simulink model "ImageBasedMdlv2"  (Simulink 9.1)
settings: Solver=VariableStepAuto  StartTime=0.0  StopTime=10.0  RelTol=1e-3
settings Model: Creator=admin  LastModifiedBy=admin
settings DataIOCC: SaveFormat=Dataset
settings OptimizationCC: LifeSpan=auto
settings DebuggingCC: UnderspecifiedInitializationDetection=Simplified  MergeDetectMultiDrivingBlocksExec=error  SFUnexpectedBacktrackingDiag=error  SFNoUnconditionalDefaultTransitionDiag=error  SFExecutionAtInitializationDiag=warning
settings HardwareCC: ProdBitPerPointer=64  ProdBitPerSizeT=64  ProdBitPerPtrDiffT=64  ProdLargestAtomicFloat=Float  ProdIntDivRoundTo=Zero  ProdEndianess=LittleEndian  ProdWordSize=64  ProdHWDeviceType=Intel->x86-64 (Windows64)
settings ModelReferenceCC: PropagateSignalLabelsOutOfModel=on
settings CodeAppCC: StateflowObjectComments=off
settings GRTTargetCC: TargetLangStandard=C99 (ISO)  CombineOutputUpdateFcns=on  GRTInterface=off
settings ConfigComp: CovMetricSettings=dwe  CovHtmlReporting=off  CovSaveCumulativeToWorkspaceVar=off  CovSaveSingleToWorkspaceVar=off  CovExternalEMLEnable=on

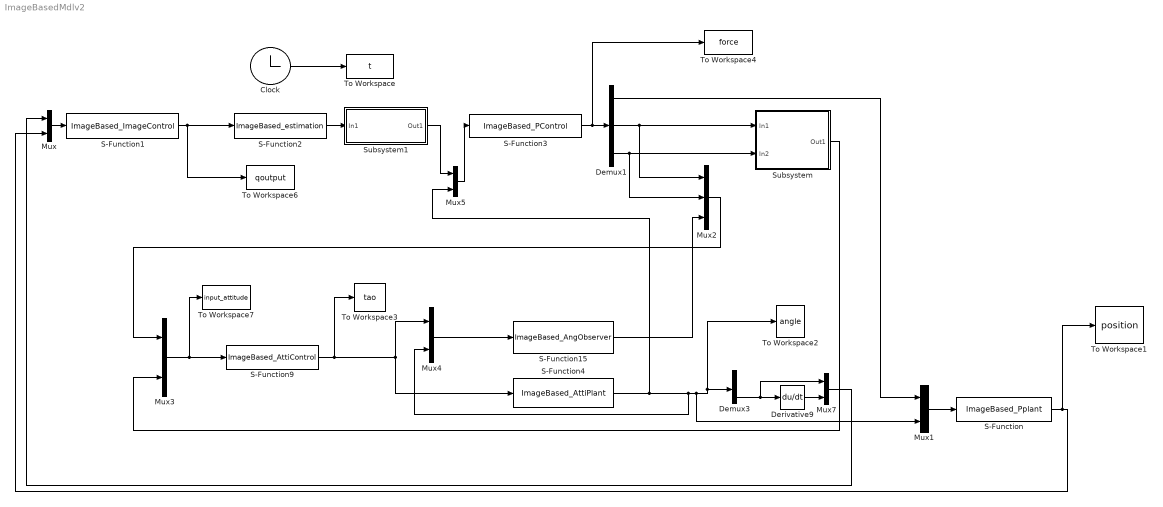
== system ImageBasedMdlv2 ==
  Clock : Clock
  Demux1 : Demux  Outputs=3
  Demux3 : Demux  Outputs=6
  Derivative9 : Derivative
  Mux{,1,3..5,7} (6 alike) : Mux  Inputs=2
  Mux2 : Mux  Inputs=3
  S-Function : S-Function  FunctionName=ImageBased_Pplant  SFunctionDeploymentMode=off  EnableBusSupport=off
  S-Function1 : S-Function  FunctionName=ImageBased_ImageControl  SFunctionDeploymentMode=off  EnableBusSupport=off
  S-Function15 : S-Function  FunctionName=ImageBased_AngObserver  SFunctionDeploymentMode=off  EnableBusSupport=off
  S-Function2 : S-Function  FunctionName=ImageBased_estimation  SFunctionDeploymentMode=off  EnableBusSupport=off
  S-Function3 : S-Function  FunctionName=ImageBased_PControl  SFunctionDeploymentMode=off  EnableBusSupport=off
  S-Function4 : S-Function  FunctionName=ImageBased_AttiPlant  SFunctionDeploymentMode=off  EnableBusSupport=off
  S-Function9 : S-Function  FunctionName=ImageBased_AttiControl  SFunctionDeploymentMode=off  EnableBusSupport=off
  Subsystem : Subsystem
  Subsystem1 : Subsystem
  To Workspace : ToWorkspace  VariableName=t  SampleTime=-1
  To Workspace1 : ToWorkspace  VariableName=position  SampleTime=-1
  To Workspace2 : ToWorkspace  VariableName=angle  SampleTime=-1
  To Workspace3 : ToWorkspace  VariableName=tao  SampleTime=-1
  To Workspace4 : ToWorkspace  VariableName=force  SampleTime=-1
  To Workspace6 : ToWorkspace  VariableName=qoutput  SampleTime=-1
  To Workspace7 : ToWorkspace  VariableName=input_attitude  SaveFormat=Timeseries  SampleTime=-1
  wires:
  S-Function3/1 -> To Workspace4/1, Demux1/1
  S-Function9/1 -> Mux4/1, S-Function4/1, To Workspace3/1
  Mux1/1 -> S-Function/1
  Mux3/1 -> To Workspace7/1, S-Function9/1
  Clock/1 -> To Workspace/1
  Derivative9/1 -> Mux7/2
  S-Function1/1 -> To Workspace6/1, S-Function2/1
  Demux3/6 -> Mux7/1, Derivative9/1
  Mux7/1 -> Mux/1
  Demux1/2 -> Mux2/1, Subsystem/1(In1)
  S-Function4/1 -> Mux5/2, Mux4/2, Mux1/2, Demux3/1, To Workspace2/1
  Mux2/1 -> Mux3/1
  Demux1/3 -> Mux2/2, Subsystem/2(In2)
  S-Function15/1 -> Mux2/3
  Mux/1 -> S-Function1/1
  S-Function2/1 -> Subsystem1/1(In1)
  S-Function/1 -> Mux/2, To Workspace1/1
  Subsystem/1(Out1) -> Mux3/2
  Demux1/1 -> Mux1/1
  Mux4/1 -> S-Function15/1
  Subsystem1/1(Out1) -> Mux5/1
  Mux5/1 -> S-Function3/1

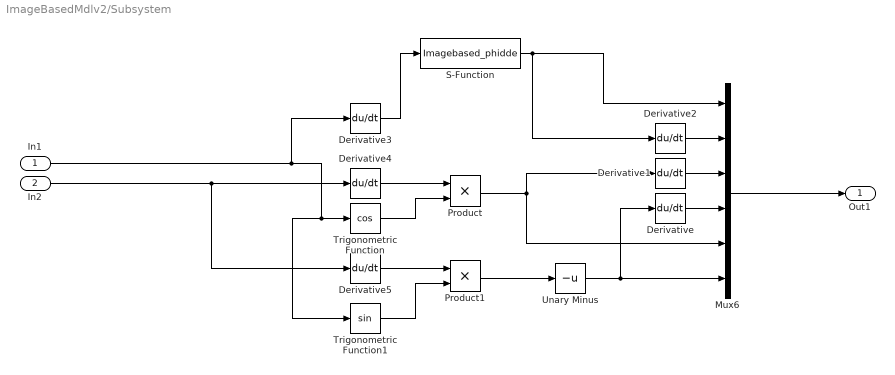
== system ImageBasedMdlv2/Subsystem ==
  In1 : Inport
  In2 : Inport  Port=2
  Derivative{,1..5} (6 alike) : Derivative
  Mux6 : Mux  Inputs=6
  Product : Product
  Product1 : Product
  S-Function : S-Function  FunctionName=Imagebased_phidde  SFunctionDeploymentMode=off  EnableBusSupport=off
  Trigonometric Function : Trigonometry  Operator=cos  OutputSignalType=real
  Trigonometric Function1 : Trigonometry
  Unary Minus : UnaryMinus
  Out1 : Outport
  wires:
  In2/1 -> Derivative5/1, Derivative4/1
  Unary Minus/1 -> Derivative/1, Mux6/6
  Trigonometric Function1/1 -> Product1/2
  Product1/1 -> Unary Minus/1
  Derivative4/1 -> Product/1
  Derivative/1 -> Mux6/4
  Product/1 -> Derivative1/1, Mux6/5
  Trigonometric Function/1 -> Product/2
  Derivative2/1 -> Mux6/2
  Derivative1/1 -> Mux6/3
  In1/1 -> Trigonometric Function1/1, Trigonometric Function/1, Derivative3/1
  Derivative5/1 -> Product1/1
  Mux6/1 -> Out1/1
  Derivative3/1 -> S-Function/1
  S-Function/1 -> Derivative2/1, Mux6/1

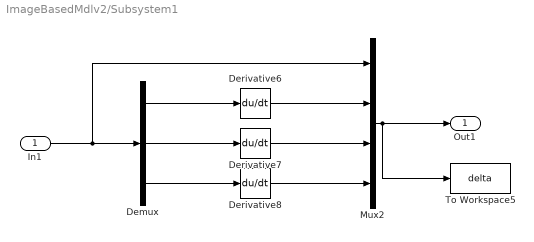
== system ImageBasedMdlv2/Subsystem1 ==
  In1 : Inport
  Demux : Demux  Outputs=3
  Derivative6 : Derivative
  Derivative7 : Derivative
  Derivative8 : Derivative
  Mux2 : Mux
  To Workspace5 : ToWorkspace  VariableName=delta  SampleTime=-1
  Out1 : Outport
  wires:
  Demux/3 -> Derivative8/1
  Derivative7/1 -> Mux2/3
  Mux2/1 -> To Workspace5/1, Out1/1
  Demux/1 -> Derivative6/1
  Derivative8/1 -> Mux2/4
  Demux/2 -> Derivative7/1
  Derivative6/1 -> Mux2/2
  In1/1 -> Mux2/1, Demux/1
